simulink library "elvio"  (R2017a)
settings: Solver=VariableStepAuto  StartTime=0.0  StopTime=10.0  RelTol=1e-3
values from neighbouring files (symbols this model uses):
  Ts = 1    [dynorun.m]
  v = [v1;v2]    [elvio_plot_scatter.m]
undefined symbols (not defined in the file or in its folder): dm, elvio_tag_from, elvio_tag_goto, energy, F, Fmax, Fmin, Freq, m, request, speed, vcur
undefined symbols (not defined in the file): containers, torque
libraries: elvio x92, simulink x6
(part 2 of 2)

== system elvio/Drive/Epicyclic ==
  vF : Inport
  Rc : Inport  Port=2
  Ch2a : elvio/Basics/Ch2a
  Ch2a1 : elvio/Basics/Ch2a
  Constant1 : Constant  Value=1/(1-a)
  Constant2 : Constant  Value=1/a
  Gearing1 : elvio/Basics/Gearing
  Gearing2 : Subsystem
  Merge v : elvio/Basics/Merge v
  Split v : elvio/Basics/Split v
  vFc : Outport
  vFs : Outport  Port=2
  tag scope: F=global
  wires:
  Ch2a1/1 -> Merge v/2
  Split v/1 -> Ch2a/1
  Split v/2 -> Ch2a1/1
  vF/1 -> Split v/1
  Merge v/1 -> [F]
  Rc/1 -> Split v/2
  Gearing1/2 -> vFc/1
  Ch2a/2 -> Gearing1/1
  Gearing1/1 -> Ch2a/2
  Constant1/1 -> Gearing1/2
  [E] -> Gearing1/3
  Gearing2/2(aF) -> Ch2a1/2
  [F2] -> Gearing2/1(F)
  Gearing2/1(av) -> vFs/1
  Constant2/1 -> Gearing2/2(a)
  Ch2a1/2 -> Gearing2/3(v')
  Ch2a/1 -> Merge v/1

== system elvio/Drive/Fixed ==
  vF : Inport
  Ch2a : elvio/Basics/Ch2a
  Constant : Constant  Value=gear
  Force Loss : elvio/Basics/Force Loss  factor=factor
  Gearing : elvio/Basics/Gearing
  vF' : Outport
  tag scope: F=global
  wires:
  Constant/1 -> Gearing/2
  Gearing/1 -> [F]
  vF/1 -> Gearing/1
  Gearing/2 -> Ch2a/1
  Ch2a/1 -> Gearing/3
  Ch2a/2 -> Force Loss/1
  Force Loss/1 -> Ch2a/2
  [E] -> Force Loss/2
  Force Loss/2 -> vF'/1

== system elvio/Drive/Gearbox ==
  vF : Inport
  1-D Table : Lookup_n-D  NumberOfTableDimensions=1  BreakpointsForDimension1=[0:6]  Table=[0.1 gears]  InternalRulePriority=Speed  RndMeth=Simplest  InputSameDT=on
  Bus Selector : BusSelector  OutputSignals=info.gear
  Ch2a : elvio/Basics/Ch2a
  Force Loss : elvio/Basics/Force Loss  factor=factor
  Gearing : elvio/Basics/Gearing
  vF' : Outport
  tag scope: Brake1=global
  wires:
  Bus Selector/1 -> 1-D Table/1  "<gear>"
  Force Loss/1 -> Ch2a/2
  Ch2a/2 -> Force Loss/1
  Gearing/2 -> Ch2a/1
  Ch2a/1 -> Gearing/3
  Gearing/1 -> [Brake1]
  1-D Table/1 -> Gearing/2
  vF/1 -> Bus Selector/1, Gearing/1
  [Gearbox1] -> Force Loss/2
  Force Loss/2 -> vF'/1

== system elvio/Drive/IVT ==
  vF : Inport
  ratio : Inport  Port=2
  Ch2a : elvio/Basics/Ch2a
  Force Loss : elvio/Basics/Force Loss  factor=factor
  Gearing : elvio/Basics/Gearing
  vF' : Outport
  tag scope: F=global
  wires:
  Force Loss/1 -> Ch2a/2
  Ch2a/2 -> Force Loss/1
  Gearing/2 -> Ch2a/1
  Ch2a/1 -> Gearing/3
  vF/1 -> Gearing/1
  Gearing/1 -> [F]
  ratio/1 -> Gearing/2
  Force Loss/2 -> vF'/1
  [E] -> Force Loss/2

== system elvio/Drive/Init ==

== system elvio/Drive/Meter ==
  vF : Inport
  Bus Selector4 : BusSelector  OutputSignals=energy
  Display : Display
  S-Function : S-Function  FunctionName=elvio_display_sfct  SFunctionDeploymentMode=off  EnableBusSupport=off
  vF' : Outport
  tag scope: F=global
  wires:
  [E] -> [F], Bus Selector4/1
  vF/1 -> vF'/1
  Bus Selector4/1 -> S-Function/1  "<energy>"
  S-Function/1 -> Display/1

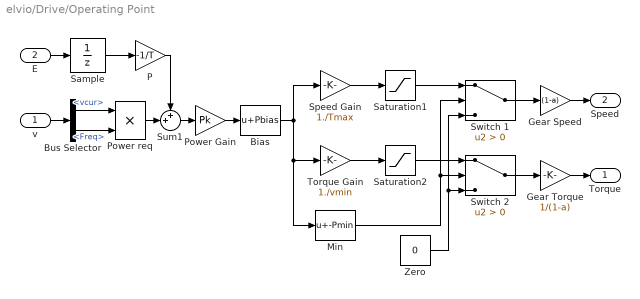
== system elvio/Drive/Operating Point ==
  v : Inport
  E : Inport  Port=2
  Bias : Bias  Bias=Pbias
  Bus Selector : BusSelector  OutputSignals=vcur,Freq
  Gear Speed : Gain  Gain=(1-a)
  Gear Torque : Gain  Gain=1/(1-a)
  Min : Bias  Bias=-Pmin
  P : Gain  Gain=-1/T
  Power Gain : Gain  Gain=Pk
  Power req : Product
  Sample : UnitDelay  SampleTime=abs(Ts)
  Saturation1 : Saturate  UpperLimit=vmax  LowerLimit=vmin
  Saturation2 : Saturate  UpperLimit=Tmax  LowerLimit=Tmin
  Speed Gain : Gain  Gain=1./Tmax
  Sum1 : Sum  Inputs=++|
  Switch 1 : Switch  Criteria=u2 > Threshold
  Switch 2 : Switch  Criteria=u2 > Threshold
  Torque Gain : Gain  Gain=1./vmin
  Zero : Constant  Value=0
  Torque : Outport
  Speed : Outport  Port=2
  wires:
  Bus Selector/2 -> Power req/2  "<Freq>"
  v/1 -> Bus Selector/1
  Gear Speed/1 -> Speed/1
  Gear Torque/1 -> Torque/1
  Bus Selector/1 -> Power req/1  "<vcur>"
  Bias/1 -> Speed Gain/1, Torque Gain/1, Min/1
  Sum1/1 -> Power Gain/1
  P/1 -> Sum1/1
  E/1 -> Sample/1
  Sample/1 -> P/1
  Power req/1 -> Sum1/2
  Power Gain/1 -> Bias/1
  Switch 1/1 -> Gear Speed/1
  Speed Gain/1 -> Saturation1/1
  Switch 2/1 -> Gear Torque/1
  Torque Gain/1 -> Saturation2/1
  Min/1 -> Switch 1/2, Switch 2/2
  Zero/1 -> Switch 2/3, Switch 1/3
  Saturation2/1 -> Switch 2/1
  Saturation1/1 -> Switch 1/1

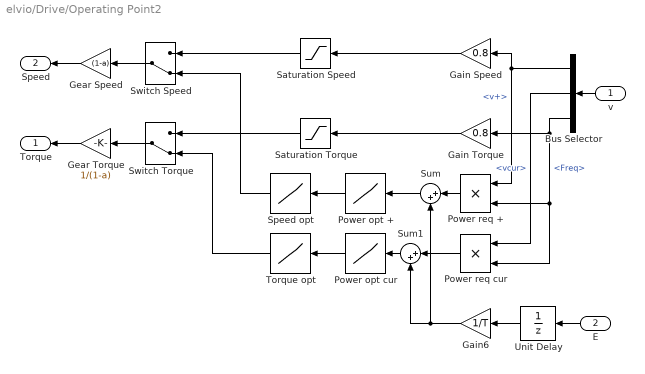
== system elvio/Drive/Operating Point2 ==
  v : Inport
  E : Inport  Port=2
  Bus Selector : BusSelector  OutputSignals=v+,vcur,Freq
  Gain Speed : Gain  Gain=0.8
  Gain Torque : Gain  Gain=0.8
  Gain6 : Gain  Gain=1/T
  Gear Speed : Gain  Gain=(1-a)
  Gear Torque : Gain  Gain=1/(1-a)
  Power opt + : Lookup_n-D  NumberOfTableDimensions=1  BreakpointsForDimension1=Preq  Table=Pice  InternalRulePriority=Speed  RndMeth=Simplest  InputSameDT=on
  Power opt cur : Lookup_n-D  NumberOfTableDimensions=1  BreakpointsForDimension1=Preq  Table=Pice  InternalRulePriority=Speed  RndMeth=Simplest  InputSameDT=on
  Power req + : Product
  Power req cur : Product
  Saturation Speed : Saturate  UpperLimit=500  LowerLimit=0
  Saturation Torque : Saturate  UpperLimit=100  LowerLimit=10
  Speed opt : Lookup_n-D  NumberOfTableDimensions=1  BreakpointsForDimension1=(Topt+1e-10).*(vopt+1e-10)  Table=vopt  ExtrapMethod=Clip  InternalRulePriority=Speed  RndMeth=Simplest  InputSameDT=on
  Sum : Sum  Inputs=|++
  Sum1 : Sum  Inputs=|++
  Switch Speed : ManualSwitch  CurrentSetting=0
  Switch Torque : ManualSwitch  CurrentSetting=0
  Torque opt : Lookup_n-D  NumberOfTableDimensions=1  BreakpointsForDimension1=(Topt+1e-10).*(vopt+1e-10)  Table=Topt  ExtrapMethod=Clip  InternalRulePriority=Speed  RndMeth=Simplest  InputSameDT=on
  Unit Delay : UnitDelay  SampleTime=abs(Ts)
  Torque : Outport
  Speed : Outport  Port=2
  wires:
  Bus Selector/1 -> Power req +/1, Gain Speed/1  "<v+>"
  Bus Selector/3 -> Power req cur/2, Power req +/2, Gain Torque/1  "<Freq>"
  v/1 -> Bus Selector/1
  Gear Speed/1 -> Speed/1
  Gear Torque/1 -> Torque/1
  Gain Speed/1 -> Saturation Speed/1
  Gain Torque/1 -> Saturation Torque/1
  Bus Selector/2 -> Power req cur/1  "<vcur>"
  Power req cur/1 -> Sum1/1
  Sum/1 -> Power opt +/1
  Speed opt/1 -> Switch Speed/2
  Torque opt/1 -> Switch Torque/2
  Power opt +/1 -> Speed opt/1
  Power opt cur/1 -> Torque opt/1
  Power req +/1 -> Sum/1
  Sum1/1 -> Power opt cur/1
  Gain6/1 -> Sum/2, Sum1/2
  Switch Speed/1 -> Gear Speed/1
  Switch Torque/1 -> Gear Torque/1
  Saturation Speed/1 -> Switch Speed/1
  Saturation Torque/1 -> Switch Torque/1
  E/1 -> Unit Delay/1
  Unit Delay/1 -> Gain6/1

== system elvio/Drive/Shaft ==
  vF : Inport
  R1 : Inport  Port=2
  Merge F : elvio/Basics/Merge F
  Split F : elvio/Basics/Split F
  vF1 : Outport
  vF2 : Outport  Port=2
  tag scope: F=global
  wires:
  Merge F/1 -> Split F/3
  [F2] -> Merge F/2
  [E] -> Merge F/1
  Split F/1 -> vF1/1
  Split F/2 -> vF2/1
  vF/1 -> Split F/1
  Merge F/2 -> [F]
  R1/1 -> Split F/2

== system elvio/Drive/Tank ==
  P : Inport
  Bus Creator : BusCreator  Inputs=2
  Bus Selector : BusSelector  OutputSignals=energy
  Ch3 : elvio/Basics/Ch1
  Minus : Gain
  Source : elvio/Basics/Source
  E : Outport
  tag scope: F=global
  wires:
  P/1 -> Ch3/2
  Ch3/2 -> [F]
  Ch3/1 -> Source/1
  Source/2 -> Bus Selector/1, Ch3/1
  Source/1 -> Bus Creator/2  "se"
  Bus Creator/1 -> E/1
  Bus Selector/1 -> Minus/1  "<energy>"
  Minus/1 -> Bus Creator/1  "energy"

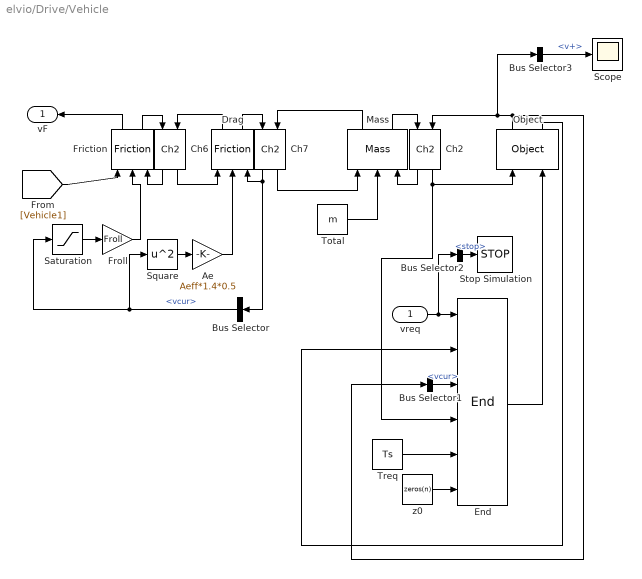
== system elvio/Drive/Vehicle ==
  vreq : Inport
  Ae : Gain  Gain=Aeff*1.4*0.5
  Bus Selector : BusSelector  OutputSignals=vcur
  Bus Selector1 : BusSelector  OutputSignals=vcur
  Bus Selector2 : BusSelector  OutputSignals=stop
  Bus Selector3 : BusSelector  OutputSignals=v+
  Ch2 : elvio/Basics/Ch2
  Ch6 : elvio/Basics/Ch2
  Ch7 : elvio/Basics/Ch2
  Drag : elvio/Basics/Friction
  End : elvio/Basics/End
  Friction : elvio/Basics/Friction
  Froll : Gain  Gain=Froll
  Mass : elvio/Basics/Mass
  Object : elvio/Basics/Object
  Saturation : Saturate  UpperLimit=1  LowerLimit=0  LinearizeAsGain=off  ZeroCross=off
  Scope : Scope
  Square : Math  Operator=square  SaturateOnIntegerOverflow=on
  Stop Simulation : Stop
  Total : Constant  Value=m  VectorParams1D=off
  Treq : Constant  Value=Ts
  z0 : Constant  Value=zeros(n)  VectorParams1D=off
  vF : Outport
  wires:
  Square/1 -> Ae/1
  Ae/1 -> Drag/2
  Total/1 -> Mass/2
  Bus Selector/1 -> Square/1, Saturation/1  "<vcur>"
  Mass/1 -> Ch7/2
  Ch7/2 -> Mass/1
  Ch7/1 -> Drag/3, Bus Selector/1
  Ch6/2 -> Drag/1
  Drag/2 -> Ch7/1
  Ch6/1 -> Friction/3
  Friction/2 -> Ch6/1
  Froll/1 -> Friction/2
  Drag/1 -> Ch6/2
  Object/2 -> End/2
  End/1 -> Object/2
  Treq/1 -> End/5
  Bus Selector3/1 -> Scope/1  "<v+>"
  z0/1 -> End/6
  Bus Selector1/1 -> End/3  "<vcur>"
  Ch2/2 -> Object/1, End/4
  Object/1 -> Bus Selector3/1, Ch2/2, Bus Selector1/1
  Mass/2 -> Ch2/1
  Ch2/1 -> Mass/3
  Friction/1 -> vF/1
  [Vehicle1] -> Friction/1
  Saturation/1 -> Froll/1
  vreq/1 -> Bus Selector2/1, End/1
  Bus Selector2/1 -> Stop Simulation/1  "<stop>"

== system elvio/Utilities/Ch0 ==
  In1 : Inport
  In2 : Inport  Port=2
  -Eps : Gain  Gain=-e
  Abs : Abs  ZeroCross=off
  Check Dynamic Range : simulink/Model Verification/Check  Dynamic Range  Description=min < u < max  enabled=on  stopWhenAssertionFail=on  export=off  icon=graphic
      settings: SourceProductName=Simulink  SourceProductBaseCode=SL
  Eps : Gain  Gain=e
  MinMax Running Resettable : simulink/Math Operations/MinMax Running Resettable  Function=max  vinit=e0
  Sum1 : Sum
  Zero : Constant  Value=0
  wires:
  MinMax Running Resettable/1 -> -Eps/1, Eps/1
  In1/1 -> Sum1/1, Abs/1
  Eps/1 -> Check Dynamic Range/1
  Abs/1 -> MinMax Running Resettable/1
  -Eps/1 -> Check Dynamic Range/2
  Sum1/1 -> Check Dynamic Range/3
  Zero/1 -> MinMax Running Resettable/2
  In2/1 -> Sum1/2

== system elvio/Utilities/Datafunction ==
  In1 : Inport
  1-D Lookup Table : Lookup_n-D  NumberOfTableDimensions=1  BreakpointsForDimension1=[0:2:10]  Table=Data  InternalRulePriority=Speed  RndMeth=Simplest  InputSameDT=on
  Out1 : Outport
  wires:
  1-D Lookup Table/1 -> Out1/1
  In1/1 -> 1-D Lookup Table/1

== system elvio/Utilities/Display ==
  In1 : Inport
  Display : Display
  wires:
  In1/1 -> Display/1

== system elvio/Utilities/Integrator ==
  dx : Inport
  x0 : Inport  Port=2
  Delay : Delay  DelayLength=1  InitialConditionSource=Input port  SampleTime=abs(Ts)
      settings: InputPortMap=u0,p4
  Product : Product
  Sum5 : Sum  Inputs=|++
  Ts : Constant  Value=Ts
  x : Outport
  x+ : Outport  Port=2
  wires:
  Sum5/1 -> Delay/1, x+/1
  Delay/1 -> Sum5/2, x/1
  Product/1 -> Sum5/1
  dx/1 -> Product/1
  Ts/1 -> Product/2
  x0/1 -> Delay/2

== system elvio/Utilities/Integrator+ ==
  dx : Inport
  x0 : Inport  Port=2
  Delay : Delay  DelayLength=1  InitialConditionSource=Input port  SampleTime=abs(Ts)
      settings: InputPortMap=u0,p4
  MinMax : MinMax  Function=max  Inputs=2
  Product : Product
  Sum5 : Sum  Inputs=|++
  Ts : Constant  Value=Ts
  Zero : Constant  Value=0
  x : Outport
  x+ : Outport  Port=2
  wires:
  x0/1 -> Delay/2
  Ts/1 -> Product/2
  dx/1 -> Product/1
  Product/1 -> Sum5/1
  Delay/1 -> x/1, Sum5/2
  MinMax/1 -> Delay/1, x+/1
  Sum5/1 -> MinMax/2
  Zero/1 -> MinMax/1

== system elvio/Utilities/Range ==
  Max : Inport
  In : Inport  Port=2
  Min : Inport  Port=3
  MinMax1 : MinMax  Inputs=2
  MinMax2 : MinMax  Function=max  Inputs=2
  Out : Outport
  wires:
  MinMax1/1 -> MinMax2/1  "F"
  In/1 -> MinMax1/1
  MinMax2/1 -> Out/1  "F"
  Min/1 -> MinMax2/2
  Max/1 -> MinMax1/2

== system elvio/Utilities/Unit ==
  Constant : Constant  Value=Value
  Unit : Gain  Gain=unitmap(unitstr)
  Out : Outport
  wires:
  Constant/1 -> Unit/1
  Unit/1 -> Out/1

== system elvio/Utilities/Variants ==
  "In1 " : Inport
  Double : Subsystem  VariantControl=Variant
  Subsystem : Subsystem  VariantControl=Variant1
  " Out1" : Outport

== system elvio/Basics/Clutch/Range ==
  Max : Inport
  In : Inport  Port=2
  Min : Inport  Port=3
  MinMax1 : MinMax  Inputs=2
  MinMax2 : MinMax  Function=max  Inputs=2
  Out : Outport
  wires:
  MinMax1/1 -> MinMax2/1  "F"
  In/1 -> MinMax1/1
  MinMax2/1 -> Out/1  "F"
  Min/1 -> MinMax2/2
  Max/1 -> MinMax1/2

== system elvio/Basics/Conversion/Power ==
  v : Inport
  F : Inport  Port=2
  Bus Creator : BusCreator  Inputs=2
  Bus Selector1 : BusSelector  OutputSignals=info
  Bus Selector2 : BusSelector  OutputSignals=vcur,v+
  Product : Product  Inputs=**
  Sum4 : Sum
  half : Gain  Gain=0.5
  P : Outport
  wires:
  Sum4/1 -> half/1
  v/1 -> Bus Selector1/1, Bus Selector2/1
  Bus Selector2/1 -> Sum4/1  "<vcur>"
  Bus Selector2/2 -> Sum4/2  "<v+>"
  Bus Selector1/1 -> Bus Creator/2  "<info>"
  Bus Creator/1 -> P/1
  Product/1 -> Bus Creator/1  "P"
  half/1 -> Product/1
  F/1 -> Product/2

== system elvio/Basics/Scale/Power ==
  v : Inport
  F : Inport  Port=2
  Bus Creator : BusCreator  Inputs=2
  Bus Selector1 : BusSelector  OutputSignals=info
  Bus Selector2 : BusSelector  OutputSignals=vcur,v+
  Product : Product  Inputs=**
  Sum4 : Sum
  half : Gain  Gain=0.5
  P : Outport
  wires:
  half/1 -> Bus Creator/1  "P"
  Bus Creator/1 -> P/1
  Bus Selector1/1 -> Bus Creator/2  "<info>"
  Bus Selector2/2 -> Sum4/2  "<v+>"
  Bus Selector2/1 -> Sum4/1  "<vcur>"
  F/1 -> Product/2
  v/1 -> Bus Selector2/1, Bus Selector1/1
  Sum4/1 -> Product/1
  Product/1 -> half/1

== system elvio/Drive/Axle/Ch4 ==
  F' : Inport
  v : Inport  Port=2
  Bus Selector1 : BusSelector  OutputSignals=info.x0
  Bus Selector2 : BusSelector  OutputSignals=Freq
  Bus Selector3 : BusSelector  OutputSignals=F
  Bus Selector4 : BusSelector  OutputSignals=energy
  Ch0 : elvio/Utilities/Ch0  e=1e-6  e0=1
  Check Static Range : simulink/Model Verification/Check  Static Range  Description=-1e-10 <= u <= 1e-10  max=1e-10  max_included=on  min=-1e-10  min_included=on  enabled=on  stopWhenAssertionFail=on  export=off  icon=graphic
      settings: SourceProductName=Simulink  SourceProductBaseCode=SL
  Integrator : elvio/Utilities/Integrator  Ts=Ts
  Power : elvio/Basics/Power
  Sum2 : Sum  Inputs=+-
  Terminator : Terminator
  v' : Outport
  F : Outport  Port=2
  wires:
  Bus Selector4/1 -> Ch0/2  "<energy>"
  Integrator/2 -> Ch0/1
  Integrator/1 -> Terminator/1
  Sum2/1 -> Check Static Range/1
  Bus Selector2/1 -> Sum2/1  "<Freq>"
  v/1 -> v'/1, Bus Selector2/1, Power/1, Bus Selector1/1
  Bus Selector1/1 -> Integrator/2  "<x0>"
  F'/1 -> Bus Selector3/1, Bus Selector4/1, F/1
  Power/1 -> Integrator/1
  Bus Selector3/1 -> Sum2/2, Power/2  "<F>"

== system elvio/Drive/Cycle/Cycle ==
  t : Inport
  Cycle : Lookup_n-D  NumberOfTableDimensions=1  BreakpointsForDimension1=[0;cumsum(data(:,1))]-1  Table=[0;data(:,2)]  InternalRulePriority=Speed  RndMeth=Simplest  InputSameDT=on
  Step : Step  Time=sum(data(:,1))  SampleTime=1  ZeroCross=off
  v : Outport
  stop : Outport  Port=2
  wires:
  Cycle/1 -> v/1
  t/1 -> Cycle/1
  Step/1 -> stop/1

== system elvio/Drive/Cycle/Hysteresis ==
  Max : Inport
  Min : Inport  Port=2
  Memory : Memory
  Range : Subsystem
  gear : Outport
  wires:
  Range/1("Out ") -> gear/1, Memory/1  "gear"
  Memory/1 -> Range/2(In)
  Max/1 -> Range/1(Max)
  Min/1 -> Range/3(Min)

== system elvio/Drive/Cycle/NEDC Shift Map ==
  Speed : Inport
  Acc : Inport  Port=2
  1-D Lookup Table1 : Lookup_n-D  NumberOfTableDimensions=1  BreakpointsForDimension1=[0 10 15 35 50 70]  Table=[1 1 2 3 4 5]  InterpMethod=Flat  InternalRulePriority=Speed  RndMeth=Simplest  InputSameDT=on
  1-D Lookup Table2 : Lookup_n-D  NumberOfTableDimensions=1  BreakpointsForDimension1=[0 10 15 35 50 70]  Table=[1 2 2 3 5 5]  InterpMethod=Flat  InternalRulePriority=Speed  RndMeth=Simplest  InputSameDT=on
  1-D Lookup Table3 : Lookup_n-D  NumberOfTableDimensions=1  BreakpointsForDimension1=[0 10 15 35 50 70]  Table=[-0.1 -1.2 -1.2 -1.2 -1.2 -1.2]  InterpMethod=Flat  InternalRulePriority=Speed  RndMeth=Simplest  InputSameDT=on
  Domain unit : SignalSpecification  Unit=km/h
  Domain unit1 : SignalSpecification  Unit=km/h
  Domain unit2 : SignalSpecification  Unit=km/h
  Sum1 : Sum  Inputs=-+|
  Switch1 : Switch
  Switch2 : Switch
  Zero : Constant  Value=0
  Upper : Outport
  Lower : Outport  Port=2
  wires:
  Switch1/1 -> Domain unit1/1  "Upper limit"
  Switch2/1 -> Domain unit2/1  "Lower limit"
  Zero/1 -> Switch1/3, Switch2/3
  1-D Lookup Table3/1 -> Sum1/1
  Acc/1 -> Sum1/2
  1-D Lookup Table1/1 -> Switch2/1
  Sum1/1 -> Switch2/2, Switch1/2
  1-D Lookup Table2/1 -> Switch1/1
  Speed/1 -> Domain unit/1
  Domain unit/1 -> 1-D Lookup Table3/1, 1-D Lookup Table1/1, 1-D Lookup Table2/1
  Domain unit1/1 -> Upper/1
  Domain unit2/1 -> Lower/1

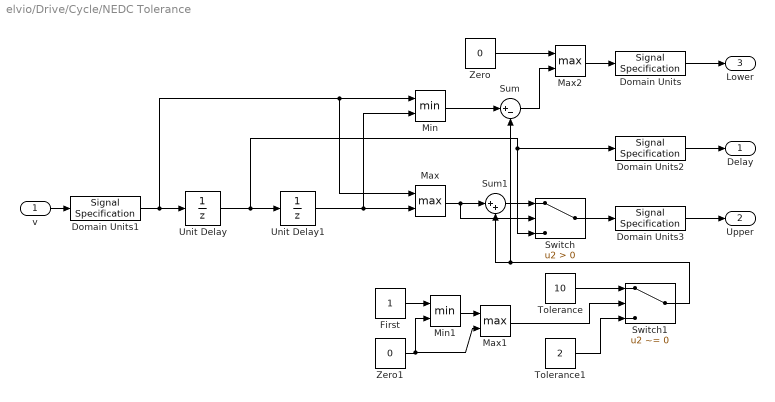
== system elvio/Drive/Cycle/NEDC Tolerance ==
  v : Inport
  Domain Units{,1..3} (4 alike) : SignalSpecification  Unit=km/h
  First : Constant
  Max : MinMax  Function=max  Inputs=2
  Max1 : MinMax  Function=max  Inputs=2
  Max2 : MinMax  Function=max  Inputs=2
  Min : MinMax  Inputs=2
  Min1 : MinMax  Inputs=2
  Sum : Sum  Inputs=|+-
  Sum1 : Sum  Inputs=|++
  Switch : Switch  Criteria=u2 > Threshold
  Switch1 : Switch  Criteria=u2 ~= 0
  Tolerance : Constant  Value=10
  Tolerance1 : Constant  Value=2
  Unit Delay : UnitDelay  SampleTime=abs(Ts)
  Unit Delay1 : UnitDelay  SampleTime=abs(Ts)
  Zero : Constant  Value=0
  Zero1 : Constant  Value=0
  Delay : Outport
  Upper : Outport  Port=2
  Lower : Outport  Port=3
  wires:
  Unit Delay1/1 -> Min/2, Max/2
  Sum/1 -> Max2/2
  v/1 -> Domain Units1/1
  Unit Delay/1 -> Unit Delay1/1, Domain Units2/1, Switch/3
  Min/1 -> Sum/1
  Tolerance1/1 -> Switch1/3
  First/1 -> Min1/1
  Zero1/1 -> Max1/2, Min1/2
  Tolerance/1 -> Switch1/1
  Switch1/1 -> Sum1/2, Sum/2
  Sum1/1 -> Switch/1
  Max1/1 -> Switch1/2
  Max/1 -> Switch/2, Sum1/1
  Min1/1 -> Max1/1
  Zero/1 -> Max2/1
  Max2/1 -> Domain Units/1
  Switch/1 -> Domain Units3/1
  Domain Units1/1 -> Unit Delay/1, Max/1, Min/1
  Domain Units/1 -> Lower/1
  Domain Units2/1 -> Delay/1
  Domain Units3/1 -> Upper/1

== system elvio/Drive/EUCycle/NEDC ==
  t : Inport
  Gear : Lookup_n-D  NumberOfTableDimensions=1  BreakpointsForDimension1=[0;cumsum(data(:,1))]  Table=[data(:,3);0]  InterpMethod=Flat  InternalRulePriority=Speed  RndMeth=Simplest  InputSameDT=on
  Signal Specification : SignalSpecification  Unit=km/hr
  Speed : Lookup_n-D  NumberOfTableDimensions=1  BreakpointsForDimension1=[0;cumsum(data(:,1))]  Table=[0;data(:,2)]  ExtrapMethod=Clip  InternalRulePriority=Speed  RndMeth=Simplest  InputSameDT=on
  Step : Step  Time=sum(data(:,1))  SampleTime=1  ZeroCross=off
  v : Outport
  g : Outport  Port=2
  stop : Outport  Port=3
  wires:
  t/1 -> Speed/1, Gear/1
  Speed/1 -> Signal Specification/1
  Signal Specification/1 -> v/1
  Gear/1 -> g/1
  Step/1 -> stop/1

== system elvio/Drive/Epicyclic/Gearing2 ==
  F : Inport
  a : Inport  Port=2
  v' : Inport  Port=3
  Bus Selector : BusSelector  OutputSignals=F,Fmax,Fmin,m,dm
  Bus Selector1 : BusSelector  OutputSignals=vcur,v+,Freq
  Bus F : BusAssignment  AssignedSignals=F,Fmax,Fmin,m,dm
  Bus v : BusAssignment  AssignedSignals=vcur,v+,Freq
  Product{1..3,5,13} (5 alike) : Product
  Product7 : Product  Inputs=***
  Product8 : Product  Inputs=/*
  Todo : Gain
  av : Outport
  aF : Outport  Port=2
  wires:
  Bus Selector/3 -> Product2/2  "<Fmin>"
  Product2/1 -> Bus F/4  "Fmin"
  Bus Selector/2 -> Product1/2  "<Fmax>"
  Product1/1 -> Bus F/3  "Fmax"
  Product5/1 -> Bus v/2  "vcur"
  Bus Selector1/3 -> Product8/2  "<Freq>"
  Product3/1 -> Bus F/2  "F"
  Product7/1 -> Bus F/5  "m"
  a/1 -> Product3/1, Product7/1, Product7/2, Product2/1, Product1/1, Product13/1, Product5/1, Product8/1
  Bus Selector/4 -> Product7/3  "<m>"
  Bus Selector/1 -> Product3/2  "<F>"
  Bus Selector/5 -> Todo/1  "<dm>"
  Bus v/1 -> av/1
  Product8/1 -> Bus v/4  "Freq"
  F/1 -> Bus F/1, Bus Selector/1
  Bus Selector1/1 -> Product5/2  "<vcur>"
  Product13/1 -> Bus v/3  "v+"
  Bus Selector1/2 -> Product13/2  "<v+>"
  v'/1 -> Bus v/1, Bus Selector1/1
  Todo/1 -> Bus F/6
  Bus F/1 -> aF/1

== system elvio/Utilities/Variants/Double ==
  "In1 " : Inport
  Gain : Gain
  " Out1" : Outport
  wires:
  "In1 "/1 -> Gain/1
  Gain/1 -> " Out1"/1

== system elvio/Utilities/Variants/Subsystem ==
  In1 : Inport
  Gain : Gain
  Out1 : Outport
  wires:
  In1/1 -> Gain/1
  Gain/1 -> Out1/1

== system elvio/Drive/Cycle/Hysteresis/Range ==
  Max : Inport
  In : Inport  Port=2
  Min : Inport  Port=3
  MinMax : MinMax  Inputs=2
  MinMax1 : MinMax  Function=max  Inputs=2
  "Out " : Outport
  wires:
  Max/1 -> MinMax/2
  MinMax/1 -> MinMax1/1  "F"
  In/1 -> MinMax/1
  Min/1 -> MinMax1/2
  MinMax1/1 -> "Out "/1  "F"
